simulink model "allModesSerial"  (R2023b)
settings: Solver=FixedStepAuto  StartTime=0.0  StopTime=10.0  FixedStep=1e-3  RelTol=1e-3  EnableMultiTasking=on
undefined symbols (not defined in the file): A0, A1, D0, D1, D10, D11, D12, D13, D2, D3, D4, D5, D6, D7, D8, D9, PTA0, PTA1, PTA2, PTB2, PTB23, PTB3, PTB9, PTC16, PTC17, PTC2, PTC3, PTC4, PTD0, PTD1, PTD2, PTD3
libraries: frdmk64flib x23, etargetslib x2, dspstat3 x1
settings Model: ExtModeTrigDuration=5  Creator=karir  LastModifiedBy=tatha
settings SolverCC: AlgebraicLoopSolver=TrustRegion
settings OptimizationCC: EnhancedBackFolding=on  PassReuseOutputArgsAs=Individual arguments  ZeroExternalMemoryAtStartup=off  ZeroInternalMemoryAtStartup=off  MaxStackSize=64  OptimizeBlockOrder=speed  DifferentSizesBufferReuse=on  OptimizationCustomize=off  EfficientTunableParamExpr=on
settings DebuggingCC: ParameterTunabilityLossMsg=error  UnconnectedInputMsg=warning  UnconnectedOutputMsg=warning  UnconnectedLineMsg=warning
settings HardwareCC: ProdBitPerPointer=32  ProdBitPerSizeT=32  ProdBitPerPtrDiffT=32  ProdLargestAtomicInteger=Long  ProdLargestAtomicFloat=Double  ProdWordSize=32  ProdHWDeviceType=ARM Compatible->ARM Cortex
settings ModelReferenceCC: EnableRefExpFcnMdlSchedulingChecks=on
settings SFSimCC: MATLABDynamicMemAlloc=off
settings RTWCC: Description=Embedded Coder  SystemTargetFile=ert.tlc  HardwareBoard=NXP FRDM-K64F  TLCOptions="-aInlineSetEventsForThisBaseRateFcn=TLC_FALSE -aSuppressMultiTaskScheduler=TLC_FALSE  -aRateBasedStepFcn=0"  TemplateMakefile=ert_default_tmf  Toolchain=GNU Tools for ARM Embedded Processors
settings CodeAppCC: ForceParamTrailComments=on  IgnoreCustomStorageClasses=off  OperatorAnnotations=on  SimulinkDataObjDesc=on  SFDataObjDesc=on  InsertBlockDesc=on

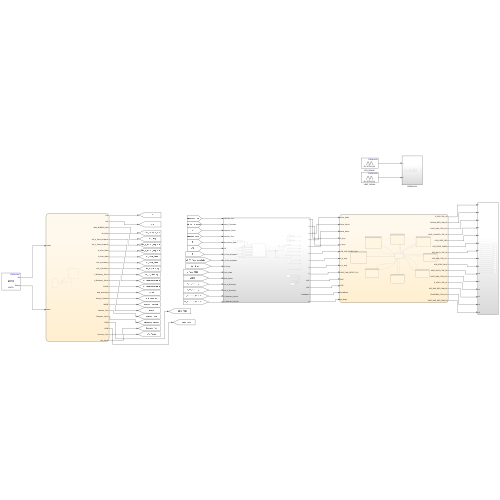
[thumbnail: Simulink's stored preview of the top-level diagram]
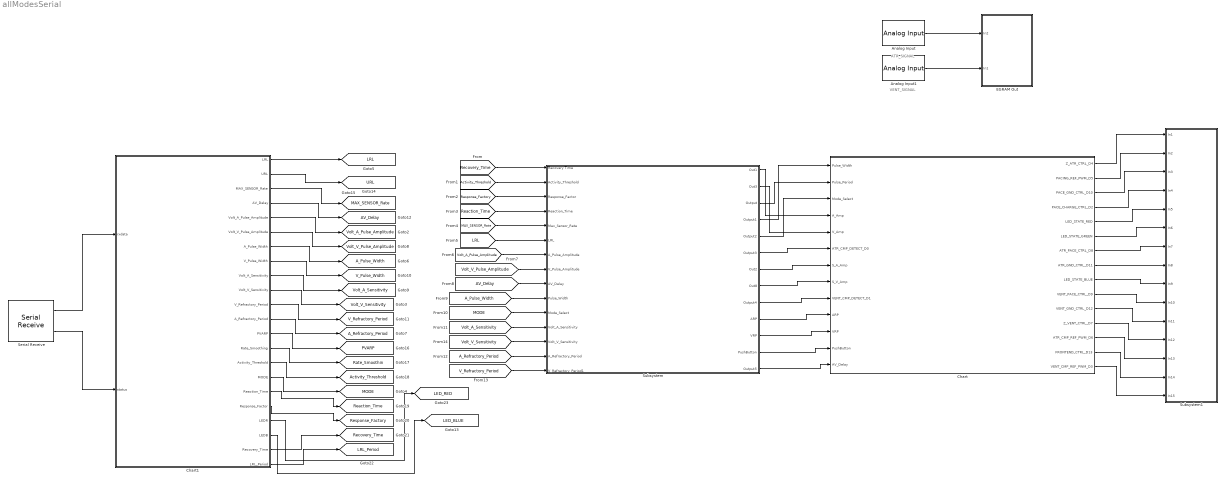
== system allModesSerial ==
  note: ATR_SIGNAL
  note: VENT_SIGNAL
  Analog Input : frdmk64flib/Analog Input  Whichpin=PTB2 (A0)  SampleTime=-1
  Analog Input1 : frdmk64flib/Analog Input  Whichpin=PTB3 (A1)  SampleTime=-1
  Chart : Stateflow chart  TreatAsAtomicUnit=on
  Chart1 : Stateflow chart  TreatAsAtomicUnit=on
      settings: PortSchema="{\"entries\":[{\"content\":{\"sides\":[{\"content\":{\"connectorIds\":[\"In1\",\"In2\"]},\"type\":\"ConnectorPlacement.EquallySpacedRectSide\",\"uuid\":\"072cf04a-3e9d-49e3-81a2-85f30e98deb0\"},{\"content\":{\"connectorIds\":[\"Out12\",\"Out14\",\"Out16\",\"Out10\",\"Out7\",\"Out1\",\"Out5\",\"Out2\",\"Out9\",\"Out8\",\"Out3\",\"Out6\",\"Out15\",\"Out18\",\"Out17\",\"Out4\",\"Out19\",\"Out20\",\"Out21\",\"Out22\",\"Out13\",\"Out11\"],\"side\":\"RIGHT\"},\"type\":\"ConnectorPlacement.EquallySpacedRectSide\",\"uuid\":\"7b2cef53-fb89-479e-8efb-56923d6ab0d7\"},{\"content\":{\"connectorIds\":[],\"side\":\"TOP\"},\"type\":\"ConnectorPlacement.EquallySpacedRectSide\",\"uuid\":\"a9a76e2c-b07f-45a0-b2fa-2ab8939b61e9\"}]},\"type\":\"ConnectorPlacement.EquallySpacedConnector\",\"uuid\":\"cead5541-bdda-40b5-b966-5757cf235cdd\"}],\"packageUris\":[\"http://schema.mathworks.com/mf0/Connector/19700101\"],\"version\":\"1.0\"}"
  EGRAM Out : Subsystem
  Serial Receive : frdmk64flib/Serial Receive  SCIModule=0  Baudrate=uint32(9600)  Parity=None  StopBits=1  HardwareFlowControl=None  ByteOrder=LittleEndian  DataType=uint8  DataLength=57  BlockingMode=off  OutputStatus=on  SampleTime=-1
  Subsystem : Subsystem
  Subsystem1 : Subsystem
  tag scope: AV_Delay=global, A_Pulse_Width=global, A_Refractory_Period=global, Activity_Threshold=global, LED_BLUE=global, LED_RED=global, LRL=global, LRL_Period=global, MAX_SENSOR_Rate=global, MODE=global, PVARP=global, Rate_Smoothin=global, Reaction_Time=global, Recovery_Time=global, Response_Factory=global, URL=global, V_Pulse_Width=global, V_Refractory_Period=global, Volt_A_Pulse_Amplitude=global, Volt_A_Sensitivity=global, Volt_V_Pulse_Amplitude=global, Volt_V_Sensitivity=global
  wires:
  Subsystem/1(Out1) -> Chart/4(A_Amp)
  Subsystem/3(Output) -> Chart/2(Pulse_Period)
  Subsystem/4(Output1) -> Chart/1(Pulse_Width)
  Subsystem/5(Output2) -> Chart/3(Mode_Select)
  Chart/1(Z_ATR_CTRL_D4) -> Subsystem1/1(In1)
  Chart/2(PACING_REF_PWM_D5) -> Subsystem1/2(In2)
  Chart/3(PACE_GND_CTRL_D10) -> Subsystem1/3(In3)
  Chart/4(PACE_CHARGE_CTRL_D2) -> Subsystem1/4(In4)
  Chart/5(LED_STATE_RED) -> Subsystem1/5(In5)
  Chart/6(LED_STATE_GREEN) -> Subsystem1/6(In6)
  Chart/7(ATR_PACE_CTRL_D8) -> Subsystem1/7(In7)
  Chart/8(ATR_GND_CTRL_D11) -> Subsystem1/8(In8)
  Chart/9(LED_STATE_BLUE) -> Subsystem1/9(In9)
  Chart/10(VENT_PACE_CTRL_D9) -> Subsystem1/10(In10)
  Chart/11(VENT_GND_CTRL_D12) -> Subsystem1/11(In11)
  Chart/12(Z_VENT_CTRL_D7) -> Subsystem1/12(In12)
  Subsystem/6(Output3) -> Chart/6(ATR_CMP_DETECT_D0)
  Subsystem/7(Out2) -> Chart/7(S_A_Amp)
  Chart/13(ATR_CMP_REF_PWM_D6) -> Subsystem1/13(In13)
  Chart/14(FRONTEND_CTRL_D13) -> Subsystem1/14(In14)
  Subsystem/9(Output4) -> Chart/9(VENT_CMP_DETECT_D1)
  Chart/15(VENT_CMP_REF_PWM_D3) -> Subsystem1/15(In15)
  Subsystem/11(VRP) -> Chart/11(VRP)
  Subsystem/12(PushButton) -> Chart/12(PushButton)
  Subsystem/10(ARP) -> Chart/10(ARP)
  Subsystem/13(Output5) -> Chart/13(AV_Delay)
  Subsystem/2(Out3) -> Chart/5(V_Amp)
  Subsystem/8(Out8) -> Chart/8(S_V_Amp)
  Serial Receive/1 -> Chart1/1(rxdata)
  Chart1/17(Activity_Threshold) -> [Activity_Threshold]
  Chart1/20(Response_Factor) -> [Response_Factory]
  Serial Receive/2 -> Chart1/2(status)
  Chart1/6(A_Refractory_Period) -> [A_Refractory_Period]
  Chart1/13(Recovery_Time) -> [Recovery_Time]
  Chart1/21(LEDR) -> [LED_RED]
  Chart1/3(V_Refractory_Period) -> [V_Refractory_Period]
  Chart1/16(MAX_SENSOR_Rate) -> [MAX_SENSOR_Rate]
  Chart1/11(LRL_Period) -> [LRL_Period]
  Chart1/1(Volt_V_Pulse_Amplitude) -> [Volt_V_Pulse_Amplitude]
  Chart1/9(Volt_A_Sensitivity) -> [Volt_A_Sensitivity]
  Chart1/10(AV_Delay) -> [AV_Delay]
  Chart1/18(Rate_Smoothing) -> [Rate_Smoothin]
  Chart1/22(LEDB) -> [LED_BLUE]
  Chart1/7(Volt_A_Pulse_Amplitude) -> [Volt_A_Pulse_Amplitude]
  Chart1/19(Reaction_Time) -> [Reaction_Time]
  Chart1/14(URL) -> [URL]
  Chart1/2(V_Pulse_Width) -> [V_Pulse_Width]
  Chart1/5(A_Pulse_Width) -> [A_Pulse_Width]
  Chart1/4(MODE) -> [MODE]
  Chart1/15(PVARP) -> [PVARP]
  Chart1/12(LRL) -> [LRL]
  Chart1/8(Volt_V_Sensitivity) -> [Volt_V_Sensitivity]
  [Recovery_Time] -> Subsystem/1(Recovery Time)
  [Activity_Threshold] -> Subsystem/2(Activity_Threshold)
  [Response_Factory] -> Subsystem/3(Response_Factor)
  [Reaction_Time] -> Subsystem/4(Reaction_Time)
  [MAX_SENSOR_Rate] -> Subsystem/5(Max_Sensor_Rate)
  [LRL] -> Subsystem/6(LRL)
  [Volt_A_Pulse_Amplitude] -> Subsystem/7(A_Pulse_Amplitude)
  [Volt_V_Pulse_Amplitude] -> Subsystem/8(V_Pulse_Amplitude)
  [AV_Delay] -> Subsystem/9(AV_Delay)
  [A_Pulse_Width] -> Subsystem/10(Pulse_Width)
  [MODE] -> Subsystem/11(Mode_Select)
  [Volt_A_Sensitivity] -> Subsystem/12(Volt_A_Sensitivity)
  [Volt_V_Sensitivity] -> Subsystem/13(Volt_V_Sensitivity)
  [A_Refractory_Period] -> Subsystem/14(A_Refractory_Period)
  [V_Refractory_Period] -> Subsystem/15(V_Refractory_Period1)
  Analog Input/1 -> EGRAM Out/1(In2)
  Analog Input1/1 -> EGRAM Out/2(In1)

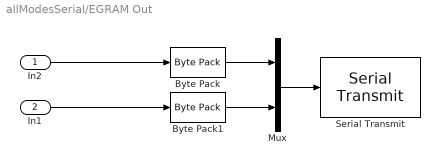
== system allModesSerial/EGRAM Out ==
  In2 : Inport
  In1 : Inport  Port=2
  Byte Pack : etargetslib/Byte Pack  datatypes={'single'}  byteAlign=1
  Byte Pack1 : etargetslib/Byte Pack  datatypes={'single'}  byteAlign=1
  Mux : Mux  Inputs=2
  Serial Transmit : frdmk64flib/Serial Transmit  SCIModule=0  Baudrate=uint32(9600)  Parity=None  StopBits=1  HardwareFlowControl=None  ByteOrder=LittleEndian  BlockingMode=on  OutputStatus=off
  wires:
  In1/1 -> Byte Pack1/1
  In2/1 -> Byte Pack/1
  Byte Pack/1 -> Mux/1
  Byte Pack1/1 -> Mux/2
  Mux/1 -> Serial Transmit/1

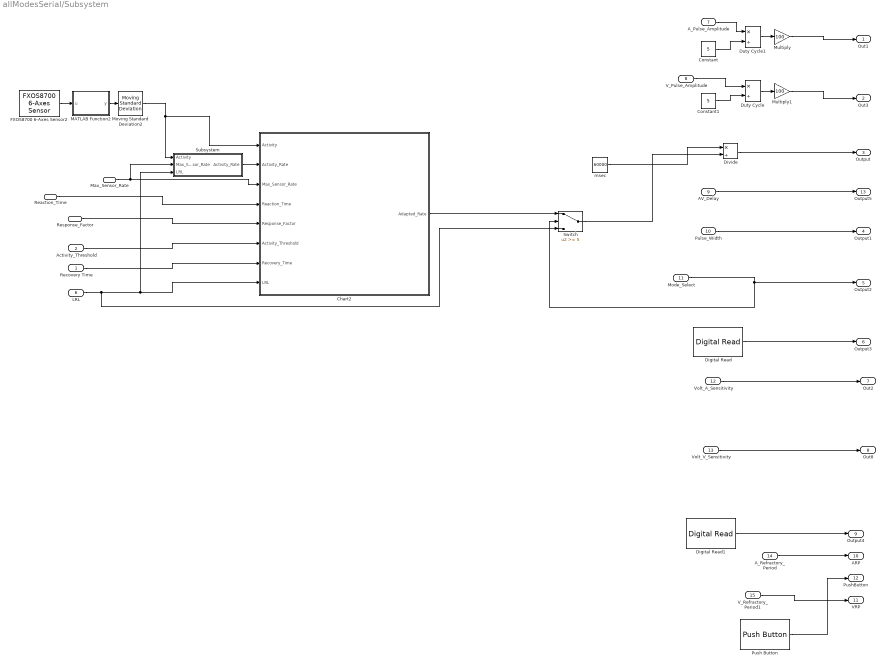
== system allModesSerial/Subsystem ==
  Recovery Time : Inport
  Activity_Threshold : Inport  Port=2
  Response_Factor : Inport  Port=3
  Reaction_Time : Inport  Port=4
  Max_Sensor_Rate : Inport  Port=5
  LRL : Inport  Port=6
  A_Pulse_Amplitude : Inport  Port=7
  V_Pulse_Amplitude : Inport  Port=8
  AV_Delay : Inport  Port=9
  Pulse_Width : Inport  Port=10
  Mode_Select : Inport  Port=11
  Volt_A_Sensitivity : Inport  Port=12
  Volt_V_Sensitivity : Inport  Port=13
  A_Refractory_Period : Inport  Port=14
  V_Refractory_Period1 : Inport  Port=15
  Chart2 : Stateflow chart  TreatAsAtomicUnit=on
  Constant : Constant  Value=5
  Constant1 : Constant  Value=5
  Digital Read : frdmk64flib/Digital Read  Whichpin=PTC16 (D0)  SampleTime=-1
  Digital Read1 : frdmk64flib/Digital Read  Whichpin=PTC17 (D1)  SampleTime=-1
  Divide : Product  Inputs=*/
  Duty Cycle : Product  Inputs=*/
  Duty Cycle1 : Product  Inputs=*/
  FXOS8700 6-Axes Sensor2 : frdmk64flib/FXOS8700 6-Axes Sensor  Activesensor=Accelerometer only  ODR=100Hz  HybridODR=400Hz  Accelfullrange=-4g to +4g  SampleTime=1/100
  MATLAB Function2 : MATLAB Function  TreatAsAtomicUnit=on
  Moving Standard Deviation2 : dspstat3/Moving Standard Deviation  Method=Sliding window  ForgettingFactorPort=off  SpecifyWindowLength=on  WindowLength=100  OverlapLength=99  AllowArbitraryInputLength=off  ForgettingFactor=0.9  SimulateUsing=Code generation
  Multiply : Gain  Gain=100
  Multiply1 : Gain  Gain=100
  Push Button : frdmk64flib/Push Button  Whichswitch=SW2  SampleTime1=-1
  Subsystem : Subsystem
  Switch : Switch  Threshold=5  SaturateOnIntegerOverflow=off  InputSameDT=off
  msec : Constant  Value=60000
  Out1 : Outport
  Out3 : Outport  Port=2
  Output : Outport  Port=3
  Output1 : Outport  Port=4
  Output2 : Outport  Port=5
  Output3 : Outport  Port=6
  Out2 : Outport  Port=7
  Out8 : Outport  Port=8
  Output4 : Outport  Port=9
  ARP : Outport  Port=10
  VRP : Outport  Port=11
  PushButton : Outport  Port=12
  Output5 : Outport  Port=13
  wires:
  msec/1 -> Divide/1
  Pulse_Width/1 -> Output1/1
  Divide/1 -> Output/1
  Digital Read/1 -> Output3/1
  Volt_A_Sensitivity/1 -> Out2/1
  Digital Read1/1 -> Output4/1
  A_Refractory_Period/1 -> ARP/1
  Push Button/1 -> PushButton/1
  FXOS8700 6-Axes Sensor2/1 -> MATLAB Function2/1(u)
  Recovery Time/1 -> Chart2/7(Recovery_Time)
  MATLAB Function2/1(y) -> Moving Standard Deviation2/1
  Moving Standard Deviation2/1 -> Chart2/1(Activity), Subsystem/1(Activity)
  Subsystem/1(Activity_Rate) -> Chart2/2(Activity_Rate)
  Chart2/1(Adapted_Rate) -> Switch/1
  Max_Sensor_Rate/1 -> Subsystem/2(Max_Sensor_Rate), Chart2/3(Max_Sensor_Rate)
  Response_Factor/1 -> Chart2/5(Response_Factor)
  Mode_Select/1 -> Switch/2, Output2/1
  Switch/1 -> Divide/2
  AV_Delay/1 -> Output5/1
  Constant/1 -> Duty Cycle1/2
  Multiply/1 -> Out1/1
  Multiply1/1 -> Out3/1
  Constant1/1 -> Duty Cycle/2
  Duty Cycle/1 -> Multiply1/1
  Duty Cycle1/1 -> Multiply/1
  Volt_V_Sensitivity/1 -> Out8/1
  Activity_Threshold/1 -> Chart2/6(Activity_Threshold)
  Reaction_Time/1 -> Chart2/4(Reaction_Time)
  LRL/1 -> Switch/3, Subsystem/3(LRL), Chart2/8(LRL)
  A_Pulse_Amplitude/1 -> Duty Cycle1/1
  V_Pulse_Amplitude/1 -> Duty Cycle/1
  V_Refractory_Period1/1 -> VRP/1

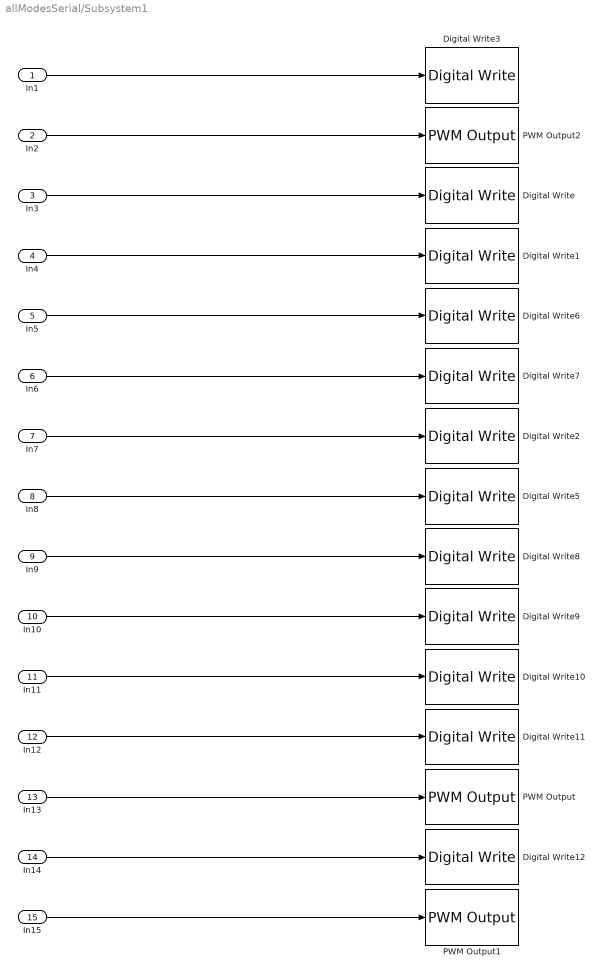
== system allModesSerial/Subsystem1 ==
  In1 : Inport
  In2 : Inport  Port=2
  In3 : Inport  Port=3
  In4 : Inport  Port=4
  In5 : Inport  Port=5
  In6 : Inport  Port=6
  In7 : Inport  Port=7
  In8 : Inport  Port=8
  In9 : Inport  Port=9
  In10 : Inport  Port=10
  In11 : Inport  Port=11
  In12 : Inport  Port=12
  In13 : Inport  Port=13
  In14 : Inport  Port=14
  In15 : Inport  Port=15
  Digital Write : frdmk64flib/Digital Write  Whichpin=PTD0 (D10)
  Digital Write1 : frdmk64flib/Digital Write  Whichpin=PTB9 (D2)
  Digital Write10 : frdmk64flib/Digital Write  Whichpin=PTD3 (D12)
  Digital Write11 : frdmk64flib/Digital Write  Whichpin=PTC3 (D7)
  Digital Write12 : frdmk64flib/Digital Write  Whichpin=PTD1 (D13)
  Digital Write2 : frdmk64flib/Digital Write  Whichpin=PTA0 (D8)
  Digital Write3 : frdmk64flib/Digital Write  Whichpin=PTB23 (D4)
  Digital Write5 : frdmk64flib/Digital Write  Whichpin=PTD2 (D11)
  Digital Write6 : frdmk64flib/Digital Write  Whichpin=RED_LED
  Digital Write7 : frdmk64flib/Digital Write  Whichpin=GREEN_LED
  Digital Write8 : frdmk64flib/Digital Write  Whichpin=BLUE_LED
  Digital Write9 : frdmk64flib/Digital Write  Whichpin=PTC4 (D9)
  PWM Output : frdmk64flib/PWM Output  Whichpin=PTC2 (D6)  InitialFrequency=2000  InitialDutyCycle=0
  PWM Output1 : frdmk64flib/PWM Output  Whichpin=PTA1 (D3)  InitialFrequency=2000  InitialDutyCycle=0
  PWM Output2 : frdmk64flib/PWM Output  Whichpin=PTA2 (D5)  InitialFrequency=2000  InitialDutyCycle=0
  wires:
  In6/1 -> Digital Write7/1
  In5/1 -> Digital Write6/1
  In1/1 -> Digital Write3/1
  In2/1 -> PWM Output2/1
  In4/1 -> Digital Write1/1
  In8/1 -> Digital Write5/1
  In7/1 -> Digital Write2/1
  In3/1 -> Digital Write/1
  In12/1 -> Digital Write11/1
  In9/1 -> Digital Write8/1
  In10/1 -> Digital Write9/1
  In11/1 -> Digital Write10/1
  In13/1 -> PWM Output/1
  In14/1 -> Digital Write12/1
  In15/1 -> PWM Output1/1

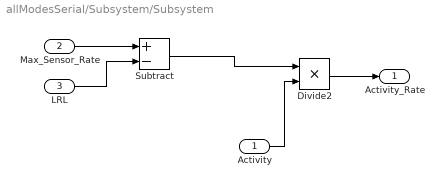
== system allModesSerial/Subsystem/Subsystem ==
  Activity : Inport
  Max_Sensor_Rate : Inport  Port=2
  LRL : Inport  Port=3
  Divide2 : Product  Inputs=**  OutDataTypeStr=uint16
  Subtract : Sum  Inputs=+-
  Activity_Rate : Outport  VectorParamsAs1DForOutWhenUnconnected=off
  wires:
  Max_Sensor_Rate/1 -> Subtract/1
  LRL/1 -> Subtract/2
  Subtract/1 -> Divide2/1
  Activity/1 -> Divide2/2
  Divide2/1 -> Activity_Rate/1

== stateflow chart allModesSerial/Chart1 ==
  state INITIAL1 [commented out]
    entry:
    LRL=60;
    URL=50;
    MAX_SENSOR_Rate=0;
    AV_Delay=20;
    Volt_A_Pulse_Amplitude=(4*100)/5;
    Volt_V_Pulse_Amplitude=(4*100)/5;
    A_Pulse_Width=10;
    V_Pulse_Width=10;
    Volt_A_Sensitivity=(4*100)/5;
    Volt_V_Sensitivity=(4*100)/5;
    V_Refractory_Period=300;
    A_Refractory_Period=300;
    PVARP=0;
    Rate_Smoothing=0;
    Activity_Threshold=0.1;
    Reaction_Time=10;
    Response_Factor=10;
    Recovery_Time;
    MODE=1;
    LRL_Period=60000/30;
  state INITIAL2 [commented out]
    entry:
    LRL=120;
    URL=50;
    MAX_SENSOR_Rate=0;
    AV_Delay=20;
    Volt_A_Pulse_Amplitude=(4*100)/5;
    Volt_V_Pulse_Amplitude=(4*100)/5;
    A_Pulse_Width=10;
    V_Pulse_Width=10;
    Volt_A_Sensitivity=(4*100)/5;
    Volt_V_Sensitivity=(4*100)/5;
    V_Refractory_Period=300;
    A_Refractory_Period=300;
    PVARP=0;
    Rate_Smoothing=0;
    Activity_Threshold=0.1;
    Reaction_Time=10;
    Response_Factor=10;
    Recovery_Time;
    MODE=1;
    LRL_Period=60000/120;
  state SET_PARAM
    entry:
    MODE=cast(rxdata(1),'uint16');
    LRL=cast(rxdata(2),'uint16');
    URL=cast(rxdata(3),'uint16');
    MAX_SENSOR_Rate=cast(rxdata(4),'uint16');
    AV_Delay=cast(rxdata(5),'uint16');
    Volt_A_Pulse_Amplitude=typecast(rxdata(6:13),'double');
    Volt_V_Pulse_Amplitude=typecast(rxdata(14:21),'double');
    A_Pulse_Width=cast(rxdata(22),'uint16');
    V_Pulse_Width=cast(rxdata(23),'uint16');
    Volt_A_Sensitivity=typecast(rxdata(24:31),'double');
    Volt_V_Sensitivity=typecast(rxdata(32:39),'double');
    V_Refractory_Period=typecast(rxdata(40:41),'uint16');
    A_Refractory_Period=typecast(rxdata(42:43),'uint16');
    PVARP=cast(rxdata(44),'uint16');
    Rate_Smoothing=cast(rxdata(45),'uint16');
    Activity_Threshold=typecast(rxdata(46:53),'double');
    Reaction_Time=cast(rxdata(54),'uint16');
    Response_Factor=cast(rxdata(55),'double');
    Recovery_Time=cast(rxdata(56),'uint16');
    LRL_Period = 60000/cast(LRL,'uint16')
    LEDR=1;
    LEDB=0;
  state INITIAL
    entry:
    LRL=60;
    URL=50;
    MAX_SENSOR_Rate=0;
    AV_Delay=20;
    Volt_A_Pulse_Amplitude=4;
    Volt_V_Pulse_Amplitude=4;
    A_Pulse_Width=10;
    V_Pulse_Width=10;
    Volt_A_Sensitivity=4;
    Volt_V_Sensitivity=4;
    V_Refractory_Period=300;
    A_Refractory_Period=300;
    PVARP=0;
    Rate_Smoothing=0;
    Activity_Threshold=0.1;
    Reaction_Time=10;
    Response_Factor=10;
    Recovery_Time=10;
    LRL_Period=10;
    MODE=1;
  state Standby
    %waiting for COM
  state ECHO_PARAM [commented out]
    entry:
    send_params();
    LEDB=1;
    LEDR=0;
    ECHO_PARAM -> ECHO_PARAM [commented out]
  INITIAL2 -> INITIAL1 [commented out] : [after(10,sec)]
  INITIAL1 -> INITIAL2 [commented out] : [after(10,sec)]
  (default) -> INITIAL
  SET_PARAM -> Standby
  (junction 44) -> SET_PARAM : [rxdata(57)==hex2dec('00')]
  (junction 43) -> Standby [order 2]
  INITIAL -> Standby
  Standby -> (junction 43) : [status==0]
  (junction 43) -> (junction 44) [order 1]
  (junction 44) -> ECHO_PARAM [commented out] : [rxdata(57)==hex2dec('01')]
  ECHO_PARAM -> Standby [commented out]
  data: Volt_V_Pulse_Amplitude output double; V_Pulse_Width output uint16; V_Refractory_Period output uint16; MODE output uint16; A_Pulse_Width output uint16; A_Refractory_Period output uint16; Volt_A_Pulse_Amplitude output double; Volt_V_Sensitivity output double; Volt_A_Sensitivity output double; AV_Delay output uint16; rxdata input uint8; status input uint8; LRL_Period output uint16; LRL output uint16; Recovery_Time output uint16; URL output uint16; PVARP output uint16; MAX_SENSOR_Rate output uint16; Activity_Threshold output double; Rate_Smoothing output uint16; Reaction_Time output uint16; Response_Factor output double; LEDR output; LEDB output

== stateflow chart allModesSerial/Chart ==
  state VOO
    state Charging
      entry:
      PACING_REF_PWM_D5 = V_Amp;
      PACE_CHARGE_CTRL_D2 = 1;
      VENT_PACE_CTRL_D9 = 0;
      VENT_GND_CTRL_D12 = 1;
      PACE_GND_CTRL_D10 = 0;
      Z_VENT_CTRL_D7 = 0;
      LED_STATE_RED = false;
      LED_STATE_BLUE = true;
    state Pacing
      entry:
      PACING_REF_PWM_D5 = V_Amp;
      PACE_CHARGE_CTRL_D2 = 0;
      VENT_PACE_CTRL_D9 = 1;
      VENT_GND_CTRL_D12 = 0;
      PACE_GND_CTRL_D10 = 1;
      Z_VENT_CTRL_D7 = 0;
      LED_STATE_RED = true;
      LED_STATE_BLUE = false;
    (default) -> VOO.Charging
    VOO.Charging -> VOO.Pacing : [after(Pulse_Period - Pulse_Width,msec)]
    VOO.Pacing -> VOO.Charging : [after(Pulse_Width,msec)]
  state VOOR
    state Charging
      entry:
      PACING_REF_PWM_D5 = V_Amp;
      PACE_CHARGE_CTRL_D2 = 1;
      VENT_PACE_CTRL_D9 = 0;
      VENT_GND_CTRL_D12 = 1;
      PACE_GND_CTRL_D10 = 0;
      Z_VENT_CTRL_D7 = 0;
      LED_STATE_RED = false;
      LED_STATE_BLUE = true;
    state Pacing
      entry:
      PACING_REF_PWM_D5 = V_Amp;
      PACE_CHARGE_CTRL_D2 = 0;
      VENT_PACE_CTRL_D9 = 1;
      VENT_GND_CTRL_D12 = 0;
      PACE_GND_CTRL_D10 = 1;
      Z_VENT_CTRL_D7 = 0;
      LED_STATE_RED = true;
      LED_STATE_BLUE = false;
    (default) -> VOOR.Charging
    VOOR.Charging -> VOOR.Pacing : [after(Pulse_Period - Pulse_Width,msec)]
    VOOR.Pacing -> VOOR.Charging : [after(Pulse_Width,msec)]
  state AOOR
    state Chambers_Paced_Charging
      entry:
      PACING_REF_PWM_D5 = A_Amp;
      PACE_CHARGE_CTRL_D2=1;
      ATR_PACE_CTRL_D8= 0;
      ATR_GND_CTRL_D11= 1;
      PACE_GND_CTRL_D10=0;
      Z_ATR_CTRL_D4=0;
      LED_STATE_RED=true;
      LED_STATE_GREEN=false;
    state pacing
      entry:
      PACING_REF_PWM_D5 = A_Amp;
      PACE_CHARGE_CTRL_D2=0;
      ATR_PACE_CTRL_D8= 1;
      ATR_GND_CTRL_D11= 0;
      PACE_GND_CTRL_D10=1;
      Z_ATR_CTRL_D4=0;
      LED_STATE_RED=false;
      LED_STATE_GREEN=true;
    (default) -> AOOR.Chambers_Paced_Charging
    AOOR.Chambers_Paced_Charging -> AOOR.pacing : [after(Pulse_Period-Pulse_Width,msec)]
    AOOR.pacing -> AOOR.Chambers_Paced_Charging : [after(Pulse_Width,msec)]
  state AOO
    state Chambers_Paced_Charging
      entry:
      PACING_REF_PWM_D5 = A_Amp;
      PACE_CHARGE_CTRL_D2=1;
      ATR_PACE_CTRL_D8= 0;
      ATR_GND_CTRL_D11= 1;
      PACE_GND_CTRL_D10=0;
      Z_ATR_CTRL_D4=0;
      LED_STATE_RED=true;
      LED_STATE_GREEN=false;
    state pacing
      entry:
      PACING_REF_PWM_D5 = A_Amp;
      PACE_CHARGE_CTRL_D2=0;
      ATR_PACE_CTRL_D8= 1;
      ATR_GND_CTRL_D11= 0;
      PACE_GND_CTRL_D10=1;
      Z_ATR_CTRL_D4=0;
      LED_STATE_RED=false;
      LED_STATE_GREEN=true;
    (default) -> AOO.Chambers_Paced_Charging
    AOO.Chambers_Paced_Charging -> AOO.pacing : [after(Pulse_Period-Pulse_Width,msec)]
    AOO.pacing -> AOO.Chambers_Paced_Charging : [after(Pulse_Width,msec)]
  state Start_State
  state VVI
    state Pacing1
      entry:
      PACING_REF_PWM_D5 = V_Amp;
      PACE_CHARGE_CTRL_D2 = 0;
      VENT_PACE_CTRL_D9 = 1;
      VENT_GND_CTRL_D12 = 0;
      PACE_GND_CTRL_D10 = 1;
      Z_VENT_CTRL_D7 = 0;
      LED_STATE_RED = true;
      LED_STATE_BLUE = false;
    state Charging_and_Sensing1
      entry:
      PACING_REF_PWM_D5 = V_Amp;
      PACE_CHARGE_CTRL_D2 = 1;
      VENT_PACE_CTRL_D9 = 0;
      VENT_GND_CTRL_D12 = 1;
      PACE_GND_CTRL_D10 = 0;
      Z_VENT_CTRL_D7 = 0;
      LED_STATE_RED = false;
      LED_STATE_BLUE = true;
      FRONTEND_CTRL_D13 = 1;
      VENT_CMP_REF_PWM_D3 = S_V_Amp;
    (default) -> VVI.Charging_and_Sensing1
    VVI.Pacing1 -> VVI.Charging_and_Sensing1 : [after(Pulse_Width,msec)]
    VVI.Charging_and_Sensing1 -> (junction 80) : after(VRP-Pulse_Width,msec)
    (junction 80) -> VVI.Pacing1 [order 2] : after(Pulse_Period-VRP,msec)[VENT_CMP_DETECT_D1 == 0 & PushButton == false]
    (junction 80) -> VVI.Charging_and_Sensing1 [order 1] : [VENT_CMP_DETECT_D1 == 1 | PushButton == true]
  state AAIR
    state Pacing
      entry:
      PACING_REF_PWM_D5 = A_Amp;
      PACE_CHARGE_CTRL_D2=0;
      ATR_PACE_CTRL_D8= 1;
      ATR_GND_CTRL_D11= 0;
      PACE_GND_CTRL_D10=1;
      Z_ATR_CTRL_D4=0;
      LED_STATE_RED=false;
      LED_STATE_GREEN=true;
    state Charging_and_Sensing
      entry:
      PACING_REF_PWM_D5 = A_Amp;
      PACE_CHARGE_CTRL_D2=1;
      ATR_PACE_CTRL_D8= 0;
      ATR_GND_CTRL_D11= 1;
      PACE_GND_CTRL_D10=0;
      Z_ATR_CTRL_D4=0;
      LED_STATE_RED=true;
      LED_STATE_GREEN=false;
      FRONTEND_CTRL_D13 = 1;
      ATR_CMP_REF_PWM_D6 = S_A_Amp;
    (default) -> AAIR.Charging_and_Sensing
    AAIR.Pacing -> AAIR.Charging_and_Sensing : after(Pulse_Width,msec)
    AAIR.Charging_and_Sensing -> (junction 147) : after(ARP-Pulse_Width, msec)
    (junction 147) -> AAIR.Pacing [order 2] : after(Pulse_Period-ARP,msec)[ATR_CMP_DETECT_D0 == 0 & PushButton == false]
    (junction 147) -> AAIR.Charging_and_Sensing [order 1] : [ATR_CMP_DETECT_D0 == 1 | PushButton == true]
  state VVIR
    state Pacing1
      entry:
      PACING_REF_PWM_D5 = V_Amp;
      PACE_CHARGE_CTRL_D2 = 0;
      VENT_PACE_CTRL_D9 = 1;
      VENT_GND_CTRL_D12 = 0;
      PACE_GND_CTRL_D10 = 1;
      Z_VENT_CTRL_D7 = 0;
      LED_STATE_RED = true;
      LED_STATE_BLUE = false;
    state Charging_and_Sensing1
      entry:
      PACING_REF_PWM_D5 = V_Amp;
      PACE_CHARGE_CTRL_D2 = 1;
      VENT_PACE_CTRL_D9 = 0;
      VENT_GND_CTRL_D12 = 1;
      PACE_GND_CTRL_D10 = 0;
      Z_VENT_CTRL_D7 = 0;
      LED_STATE_RED = false;
      LED_STATE_BLUE = true;
      FRONTEND_CTRL_D13 = 1;
      VENT_CMP_REF_PWM_D3 = S_V_Amp;
    (default) -> VVIR.Charging_and_Sensing1
    VVIR.Pacing1 -> VVIR.Charging_and_Sensing1 : [after(Pulse_Width,msec)]
    VVIR.Charging_and_Sensing1 -> (junction 120) : after(VRP-Pulse_Width,msec)
    (junction 120) -> VVIR.Pacing1 [order 2] : after(Pulse_Period-VRP,msec)[VENT_CMP_DETECT_D1 == 0 & PushButton == false]
    (junction 120) -> VVIR.Charging_and_Sensing1 [order 1] : [VENT_CMP_DETECT_D1 == 1 | PushButton == true]
  state AAI
    state Pacing
      entry:
      PACING_REF_PWM_D5 = A_Amp;
      PACE_CHARGE_CTRL_D2=0;
      ATR_PACE_CTRL_D8= 1;
      ATR_GND_CTRL_D11= 0;
      PACE_GND_CTRL_D10=1;
      Z_ATR_CTRL_D4=0;
      LED_STATE_RED=false;
      LED_STATE_GREEN=true;
    state Charging_and_Sensing
      entry:
      PACING_REF_PWM_D5 = A_Amp;
      PACE_CHARGE_CTRL_D2=1;
      ATR_PACE_CTRL_D8= 0;
      ATR_GND_CTRL_D11= 1;
      PACE_GND_CTRL_D10=0;
      Z_ATR_CTRL_D4=0;
      LED_STATE_RED=true;
      LED_STATE_GREEN=false;
      FRONTEND_CTRL_D13 = 1;
      ATR_CMP_REF_PWM_D6 = S_A_Amp;
    (default) -> AAI.Charging_and_Sensing
    AAI.Pacing -> AAI.Charging_and_Sensing : after(Pulse_Width,msec)
    AAI.Charging_and_Sensing -> (junction 90) : after(ARP-Pulse_Width, msec)
    (junction 90) -> AAI.Pacing [order 2] : after(Pulse_Period-ARP,msec)[ATR_CMP_DETECT_D0 == 0 & PushButton == false]
    (junction 90) -> AAI.Charging_and_Sensing [order 1] : [ATR_CMP_DETECT_D0 == 1 | PushButton == true]
  Start_State -> VOOR [order 1] : [Mode_Select == 6 ]
  Start_State -> VOO [order 5] : [Mode_Select == 2 ]
  VOO -> Start_State : [Mode_Select ~= 2 ]
  VOOR -> Start_State : [Mode_Select ~= 6 ]
  (default) -> AOOR [order 2] : [Mode_Select == 5  ]
  AOOR -> Start_State : [Mode_Select ~= 5  ]
  (default) -> Start_State [order 1]
  VVI -> Start_State : [Mode_Select ~= 4 ]
  Start_State -> VVI [order 7] : [Mode_Select == 4]
  AOO -> Start_State : [Mode_Select ~= 1]
  Start_State -> AOO [order 4] : [Mode_Select == 1]
  VVIR -> Start_State : [Mode_Select ~= 8]
  Start_State -> VVIR [order 2] : [Mode_Select == 8 ]
  AAIR -> Start_State : [Mode_Select ~= 7 ]
  Start_State -> AAIR [order 3] : [Mode_Select == 7 ]
  AAI -> Start_State : [Mode_Select ~= 3]
  Start_State -> AAI [order 6] : [Mode_Select == 3]
  data: Z_ATR_CTRL_D4 output; PACING_REF_PWM_D5 output; PACE_GND_CTRL_D10 output; PACE_CHARGE_CTRL_D2 output; LED_STATE_RED output; LED_STATE_GREEN output; ATR_PACE_CTRL_D8 output; ATR_GND_CTRL_D11 output; Pulse_Width input; Pulse_Period input; Mode_Select input; A_Amp input; V_Amp input; LED_STATE_BLUE output; VENT_PACE_CTRL_D9 output; VENT_GND_CTRL_D12 output; Z_VENT_CTRL_D7 output; ATR_CMP_REF_PWM_D6 output; ATR_CMP_DETECT_D0 input; S_A_Amp input; S_V_Amp input; FRONTEND_CTRL_D13 output; VENT_CMP_DETECT_D1 input; ARP input; VENT_CMP_REF_PWM_D3 output; VRP input; PushButton input; AV_Delay input

== stateflow chart allModesSerial/Subsystem/Chart2 ==
  state Activity_Rate
  state Up
    entry:
    Time = 0;
    during:
    Adapted_Rate = Response_Factor*(Time/Reaction_Time)/(1+(Time/Reaction_Time)*(Response_Factor-1))*Activity_Rate + LRL;
    Time = Time + 1/1000;
    exit:
    Time = 0;
  state Max
    entry:
    Adapted_Rate = Max_Sensor_Rate;
  state Down
    entry:
    Time = 0;
    Rate_Diff = Adapted_Rate - LRL;
    during:
    Adapted_Rate = Adapted_Rate - (Rate_Diff/Recovery_Time)*Time;
    Time = Time + 1/1000;
    exit:
    Time = 0;
  state Start
    entry:
    Adapted_Rate = LRL;
  state Min
  Up -> Activity_Rate [order 2] : [Adapted_Rate>=Activity_Rate+LRL]
  Up -> Up [order 3] : [Time >= Reaction_Time]{Time = 0}
  Activity_Rate -> Down [order 2] : [Activity < Activity_Threshold]
  Activity_Rate -> Up [order 1] : [Activity >= Activity_Threshold]
  Up -> Max [order 1] : [Adapted_Rate >= Max_Sensor_Rate]
  Min -> Up : [Activity >= Activity_Threshold]
  Max -> Down : [Activity < Activity_Threshold]
  Up -> Down [order 4] : [Activity < Activity_Threshold]
  Down -> Up [order 1] : [Activity >= Activity_Threshold]
  (default) -> Start
  Start -> Down
  Down -> Min [order 2] : [Adapted_Rate == LRL]
  Down -> Down [order 3] : [Time >= Recovery_Time]{Time = 0}
  data: Activity input double; Activity_Rate input; Adapted_Rate output uint16; Max_Sensor_Rate input uint16; Reaction_Time input uint16; Response_Factor input double; Activity_Threshold input double; Recovery_Time input uint16; LRL input uint16; Rate_Diff local uint16; Time local double

== matlab function allModesSerial/Subsystem/MATLAB Function2 ==
  data: u input; y output
function y = fcn(u)
y = sqrt(u(1)^2+u(2)^2+u(3)^2);
